simulink model "IJAM_simulink"  (R2021a)
settings: Solver=FixedStepAuto  StartTime=Tstart  StopTime=Tsim  FixedStep=step  RelTol=1e-3
values from neighbouring files (symbols this model uses):
  a = par_gs_inv4(5)    [JAM_simulink.m]
  alpha = par_gs_inv4(4)    [JAM_simulink.m]
  c = par_gs_inv4(3)    [JAM_simulink.m]
  Hmax = max(H_35H300)    [JAM_simulink.m]
  Hsimmax = 1.4195e+03    (= 1419.5)    [JAM_simulink.m]
  k = par_gs_inv4(2)    [JAM_simulink.m]
  Ms = par_gs_inv4(1)    [JAM_simulink.m]
  mu0 = 4*pi*10^-7    (= 1.25663706144e-06)    [JAM_simulink.m]
libraries: simulink x1
settings Model: Creator=UTENTE  LastModifiedBy=UTENTE
settings SolverCC: ZeroCrossControl=DisableAll

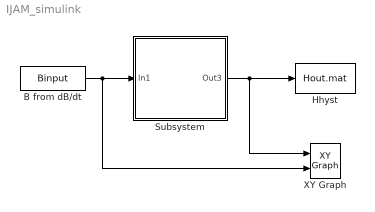
== system IJAM_simulink ==
  "B from dB/dt " : FromWorkspace  VariableName=Binput  OutDataTypeStr=double
  Hhyst : ToFile  Filename=Hout.mat  MatrixName=Hsim  SampleTime=1
  Subsystem : Subsystem
      mask Display: image('images.png'); % Use "Edit Image" on toolstrip to change.
  XY Graph : simulink/Sinks/XY Graph  xmin=-1500  xmax=1500  ymin=-1.5  ymax=1.5  st=-1
  wires:
  "B from dB/dt "/1 -> XY Graph/2, Subsystem/1(In1)
  Subsystem/1(Out3) -> XY Graph/1, Hhyst/1

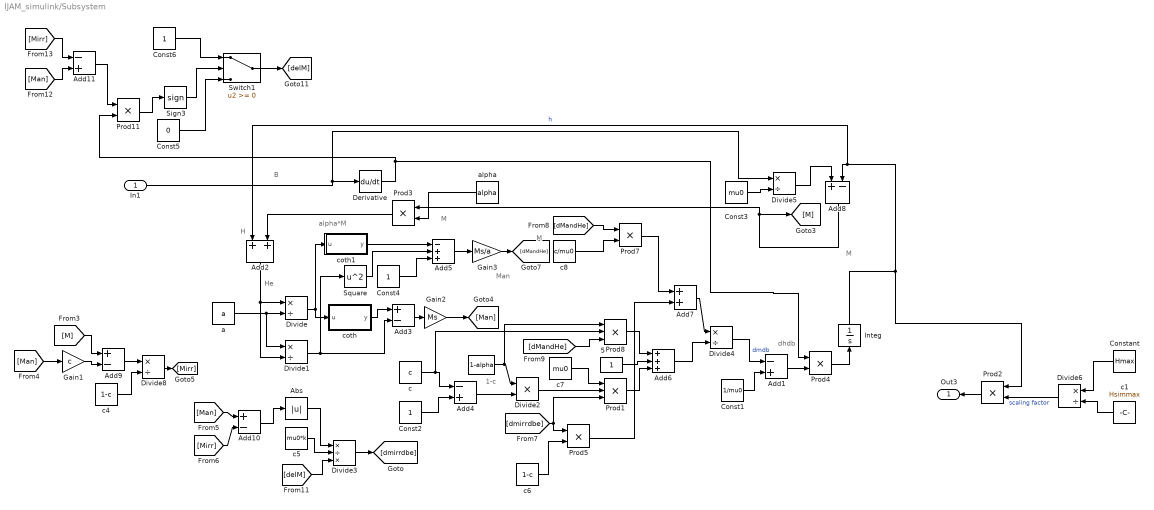
== system IJAM_simulink/Subsystem ==
  note: M
  note: B
  note: M
  note: Man
  note: 1-c
  note: dhdb
  note: H
  note: alpha*M
  note: M
  note: He
  In1 : Inport
  " " : Constant  Value=1-alpha
  5 : Constant
  Abs : Abs
  Add1 : Sum  Inputs=-+
  Add{3,8..10} (4 alike) : Sum  Inputs=+-
  Add11 : Sum  Inputs=-+
  Add2 : Sum
  Add4 : Sum  Inputs=-+
  Add5 : Sum  Inputs=-++
  Add6 : Sum  Inputs=+++
  Add7 : Sum
  Const1 : Constant  Value=1/mu0
  Const2 : Constant
  Const3 : Constant  Value=mu0
  Const4 : Constant
  Const5 : Constant  Value=0
  Const6 : Constant
  Constant : Constant  Value=Hmax
  Derivative : Derivative
  Divide{,1,4..6,8} (6 alike) : Product  Inputs=*/
  Divide2 : Product  Inputs=**
  Divide3 : Product  Inputs=*/*
  Gain1 : Gain  Gain=c
  Gain2 : Gain  Gain=Ms
  Gain3 : Gain  Gain=Ms/a
  Integ : Integrator
  Prod1 : Product  Inputs=3
  Prod{2..5,7,11} (6 alike) : Product
  Prod8 : Product  Inputs=3
  Sign3 : Signum
  Square : Math  Operator=square  SaturateOnIntegerOverflow=on
  Switch1 : Switch
  a : Constant  Value=a
  alpha : Constant  Value=alpha
  c : Constant  Value=c
  c1 : Constant  Value=Hsimmax
  c4 : Constant  Value=1-c
  c5 : Constant  Value=mu0*k
  c6 : Constant  Value=1-c
  c7 : Constant  Value=mu0
  c8 : Constant  Value=c/mu0
  coth : MATLAB Function  TreatAsAtomicUnit=on
  coth1 : MATLAB Function  TreatAsAtomicUnit=on
  Out3 : Outport
  wires:
  Prod1/1 -> Add6/3
  Add2/1 -> Divide/1, Divide1/2
  Gain2/1 -> [Man]
  Const3/1 -> Divide5/2
  Const6/1 -> Switch1/1
  [dmirrdbe] -> Prod1/3, Prod5/1
  Prod7/1 -> Add7/1
  " "/1 -> Prod8/1, Divide2/1
  Divide1/1 -> Square/1, Add3/2
  c7/1 -> Prod1/1
  Gain1/1 -> Add9/2
  Divide/1 -> coth1/1(u), coth/1(u)
  Add11/1 -> Prod11/1
  In1/1 -> Divide5/1, Derivative/1
  c5/1 -> Divide3/2
  c/1 -> Prod8/2, Add4/1
  c6/1 -> Prod5/2
  alpha/1 -> Prod3/2
  Prod3/1 -> Add2/2
  c8/1 -> Prod7/2
  Divide5/1 -> Add8/1
  Add6/1 -> Divide4/2
  [M] -> Add9/1
  Prod8/1 -> Add6/1
  Derivative/1 -> Prod4/1, Prod11/2
  [Mirr] -> Add10/2
  Add10/1 -> Abs/1
  Const1/1 -> Add1/2
  a/1 -> Divide1/1, Divide/2
  Prod11/1 -> Sign3/1
  Const2/1 -> Add4/2
  Sign3/1 -> Switch1/2
  Add1/1 -> Prod4/2
  Gain3/1 -> [dMandHe]
  Divide8/1 -> [Mirr]
  Switch1/1 -> [delM]
  Square/1 -> Add5/2
  [Man] -> Add11/2
  [delM] -> Divide3/3
  coth/1(y) -> Add3/1
  [Mirr] -> Add11/1
  Const4/1 -> Add5/3
  coth1/1(y) -> Add5/1
  Prod4/1 -> Integ/1
  Add8/1 -> [M], Prod3/1
  Add3/1 -> Gain2/1
  [dMandHe] -> Prod7/1
  Abs/1 -> Divide3/1
  Add4/1 -> Divide2/2
  [Man] -> Gain1/1
  Add7/1 -> Divide4/1
  Prod5/1 -> Add7/2
  [dMandHe] -> Prod8/3
  5/1 -> Add6/2
  Add9/1 -> Divide8/1
  Integ/1 -> Prod2/1, Add2/1, Add8/2  "h"
  Divide2/1 -> Prod1/2
  Add5/1 -> Gain3/1
  Divide4/1 -> Add1/1  "dmdb"
  Const5/1 -> Switch1/3
  Divide3/1 -> [dmirrdbe]
  [Man] -> Add10/1
  c4/1 -> Divide8/2
  Divide6/1 -> Prod2/2  "scaling factor"
  Constant/1 -> Divide6/1
  c1/1 -> Divide6/2
  Prod2/1 -> Out3/1

== matlab function IJAM_simulink/Subsystem/coth ==
  data: u input; y output
function y = cotan(u)

y = coth(u);

== matlab function IJAM_simulink/Subsystem/coth1 ==
  data: u input; y output
function y = cot2(u)

y = coth(u)^2;
